simulink model "hpt_dual_dcpool"  (R2025a)
settings: Solver=ode23tb  StartTime=0.0  StopTime=0.4  RelTol=1e-3
libraries: spsSeriesRLCBranchLib x5, spsGroundLib x2, spsControlledCurrentSourceLib x2, spsVoltageMeasurementLib x2, spsCurrentMeasurementLib x1, spspowerguiLib x1
settings Model: Creator=m1391  LastModifiedBy=m1391

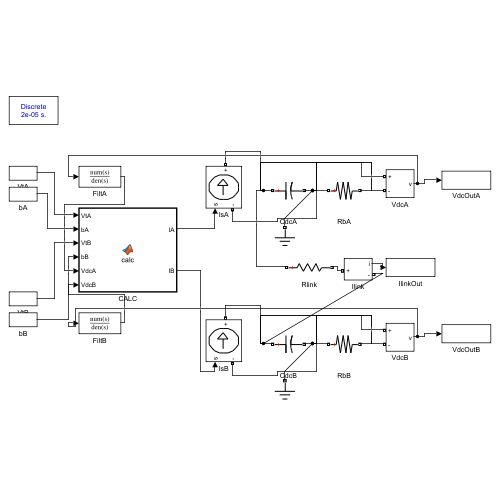
[thumbnail: Simulink's stored preview of the top-level diagram]
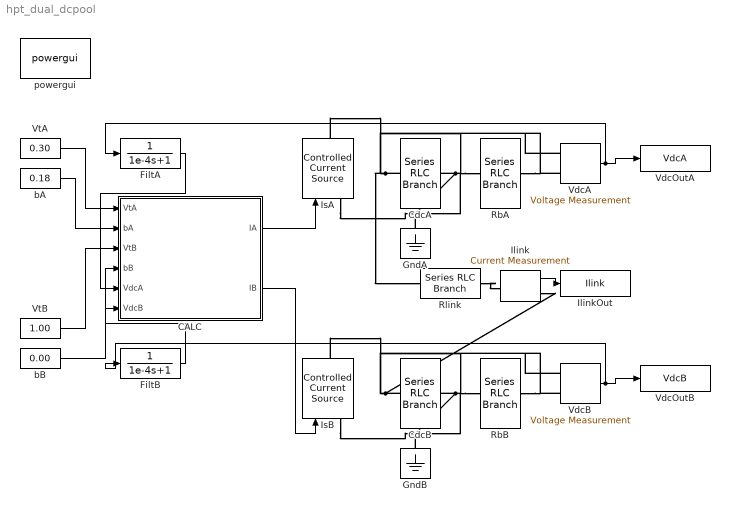
== system hpt_dual_dcpool ==
  CALC : MATLAB Function  TreatAsAtomicUnit=on
  CdcA : spsSeriesRLCBranchLib/Series RLC Branch  LConnTagsString=__new0  RConnTagsString=__new0  BranchType=C  Resistance=1  Inductance=1e-3  SetiL0=off  InitialCurrent=0  Capacitance=0.0022  Setx0=on  InitialVoltage=800  Measurements=None
  CdcB : spsSeriesRLCBranchLib/Series RLC Branch  LConnTagsString=__new0  RConnTagsString=__new0  BranchType=C  Resistance=1  Inductance=1e-3  SetiL0=off  InitialCurrent=0  Capacitance=0.0022  Setx0=on  InitialVoltage=800  Measurements=None
  FiltA : TransferFcn  Denominator=[1e-4 1]
  FiltB : TransferFcn  Denominator=[1e-4 1]
  GndA : spsGroundLib/Ground  LConnTagsString=a
  GndB : spsGroundLib/Ground  LConnTagsString=a
  Ilink : spsCurrentMeasurementLib/Current Measurement  PhasorSimulation=off  OutputType=Complex  PSBequivalent=0
  IlinkOut : ToWorkspace  VariableName=Ilink  SampleTime=2e-05
  IsA : spsControlledCurrentSourceLib/Controlled Current Source  Initialize=on  Source_Type=AC  Amplitude=0  Phase=0  Frequency=0  Measurements=None
  IsB : spsControlledCurrentSourceLib/Controlled Current Source  Initialize=on  Source_Type=AC  Amplitude=0  Phase=0  Frequency=0  Measurements=None
  RbA : spsSeriesRLCBranchLib/Series RLC Branch  LConnTagsString=__new0  RConnTagsString=__new0  BranchType=R  Resistance=100000  Inductance=1e-3  SetiL0=off  InitialCurrent=0  Capacitance=1e-6  Setx0=off  InitialVoltage=0  Measurements=None
  RbB : spsSeriesRLCBranchLib/Series RLC Branch  LConnTagsString=__new0  RConnTagsString=__new0  BranchType=R  Resistance=100000  Inductance=1e-3  SetiL0=off  InitialCurrent=0  Capacitance=1e-6  Setx0=off  InitialVoltage=0  Measurements=None
  Rlink : spsSeriesRLCBranchLib/Series RLC Branch  LConnTagsString=__new0  RConnTagsString=__new0  BranchType=R  Resistance=0.5  Inductance=1e-3  SetiL0=off  InitialCurrent=0  Capacitance=1e-6  Setx0=off  InitialVoltage=0  Measurements=None
  VdcA : spsVoltageMeasurementLib/Voltage Measurement  PhasorSimulation=off  OutputType=Complex  PSBequivalent=0
  VdcB : spsVoltageMeasurementLib/Voltage Measurement  PhasorSimulation=off  OutputType=Complex  PSBequivalent=0
  VdcOutA : ToWorkspace  VariableName=VdcA  SampleTime=2e-05
  VdcOutB : ToWorkspace  VariableName=VdcB  SampleTime=2e-05
  VtA : Constant  Value=0.30
  VtB : Constant  Value=1.00
  bA : Constant  Value=0.18
  bB : Constant  Value=0.00
  powergui : spspowerguiLib/powergui  Priority=1  SimulationMode=Discrete  SampleTime=2e-05  frequency=60  Iterations=50  frequencyindice=60  Pbase=100e6  ErrMax=1e-4  UnitsV=kV  UnitsW=MW  buscounter=0  FunctionMessages=off  echomessages=off  EnableUseOfTLC=off  CurrentSourceSwitches=off  DisableSnubberDevices=off  DisableRonSwitches=off  DisableVfSwitches=off  DisplayEquations=off  AutomaticDiscreteSolvers=off  SolverType=Tustin/Backward Euler (TBE)  Interpol=off  ExternalGateDelay=off  methode=off  Ts=100  x0status=blocks  SPID=on  SwTol=0  HookPort=off  NonlinearTolerance=1e-4  nMaxIteration=100  ContinueOnMaxIteration=off  RestoreLinks=warning  ResistiveCurrentMeasurement=off  Frange=[0:2:500]  Ylog=off  Xlog=on  ShowGrid=off  save=off  variable=ZData  structure=0  ZoomFFT=off  StartTime=0.0  cycles=1  DisplayStyle=1  fundamental=60  FreqAxis=off  MaxFrequency=1000  frequencyindicesteady=1  RmsSteady=1  display=off
  wires:
  VtA/1 -> CALC/1(VtA)
  bA/1 -> CALC/2(bA)
  VtB/1 -> CALC/3(VtB)
  bB/1 -> CALC/4(bB)
  VdcA/1 -> FiltA/1, VdcOutA/1
  FiltA/1 -> CALC/5(VdcA)
  VdcB/1 -> FiltB/1, VdcOutB/1
  FiltB/1 -> CALC/6(VdcB)
  CALC/1(IA) -> IsA/1
  CALC/2(IB) -> IsB/1
  Ilink/1 -> IlinkOut/1
  connections:
  RbA/LConn1 -- CdcA/LConn1 -- IsA/RConn1 -- VdcA/LConn1 -- Rlink/LConn1
  RbA/RConn1 -- IsA/LConn1 -- VdcA/LConn2 -- CdcA/RConn1 -- GndA/LConn1
  RbB/LConn1 -- CdcB/LConn1 -- IsB/RConn1 -- VdcB/LConn1 -- Ilink/RConn1
  RbB/RConn1 -- IsB/LConn1 -- VdcB/LConn2 -- CdcB/RConn1 -- GndB/LConn1
  Rlink/RConn1 -- Ilink/LConn1

== matlab function hpt_dual_dcpool/CALC ==
  data: VtA input; IA output; bA input; VtB input; bB input; VdcA input; VdcB input; IB output
function [IA,IB] = calc(VtA,bA,VtB,bB,VdcA,VdcB)
%#codegen
Pb=400e3; idav=0.28; Kp=20; Vref=800;
va=max(50,VdcA); vb=max(50,VdcB);
ImaxA=max(0,VtA)*idav*Pb/va; ImaxB=max(0,VtB)*idav*Pb/vb;
IinA=min(ImaxA, max(0, Kp*(Vref-va)));
IinB=min(ImaxB, max(0, Kp*(Vref-vb)));
IseA=max(0,bA)*1.9*Pb/Vref; IseB=max(0,bB)*1.9*Pb/Vref;
IA=IinA-IseA; IB=IinB-IseB;
